simulink model "COUNTERdown"  (R2016a)
settings: Solver=FixedStepDiscrete  StartTime=0.0  StopTime=10.0  RelTol=1e-3
model workspace (MAT data in the model file):
  cs : Simulink.ConfigSet (value not decoded)
settings Model: Creator=LEGION  LastModifiedBy=LEGION
settings RTWCC: GenCodeOnly=on

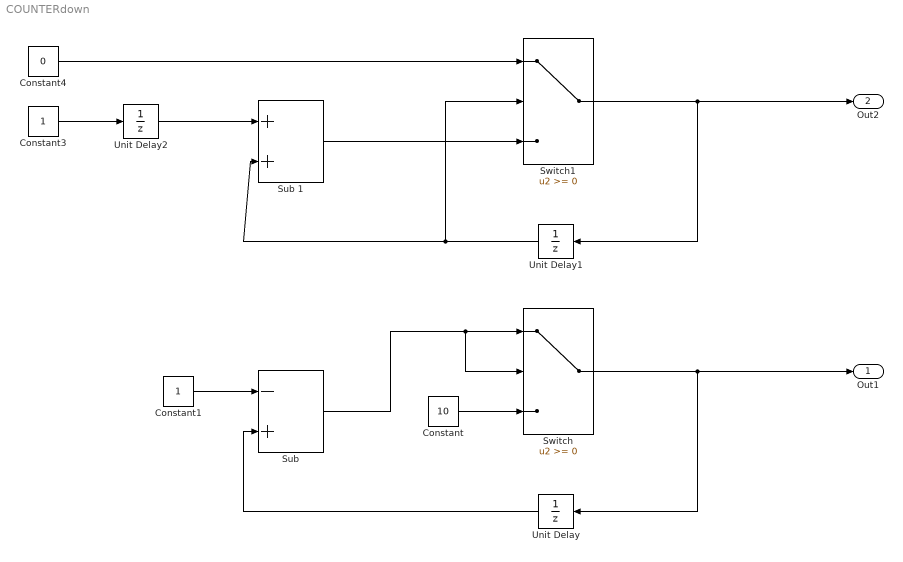
== system COUNTERdown ==
  Constant : Constant  Value=10
  Constant1 : Constant
  Constant3 : Constant
  Constant4 : Constant  Value=0
  "Sub " : Sum  Inputs=-+
  Sub 1 : Sum
  Switch : Switch
  Switch1 : Switch
  Unit Delay : UnitDelay  SampleTime=-1
  Unit Delay1 : UnitDelay  SampleTime=-1
  Unit Delay2 : UnitDelay  SampleTime=-1
  Out1 : Outport
  Out2 : Outport  Port=2
  wires:
  Switch/1 -> Out1/1, Unit Delay/1
  Unit Delay/1 -> "Sub "/2
  Constant1/1 -> "Sub "/1
  "Sub "/1 -> Switch/2, Switch/1
  Constant/1 -> Switch/3
  Switch1/1 -> Out2/1, Unit Delay1/1
  Unit Delay1/1 -> Switch1/2, Sub 1/2
  Constant4/1 -> Switch1/1
  Constant3/1 -> Unit Delay2/1
  Unit Delay2/1 -> Sub 1/1
  Sub 1/1 -> Switch1/3
